simulink model "LowPassRC_Filter"  (R2021a)
settings: Solver=FixedStepAuto  StartTime=0.0  StopTime=10.0  FixedStep=0.0001  RelTol=1e-3
libraries: simulink x1
settings Model: Creator=F Octopus The Grey  LastModifiedBy=F Octopus The Grey

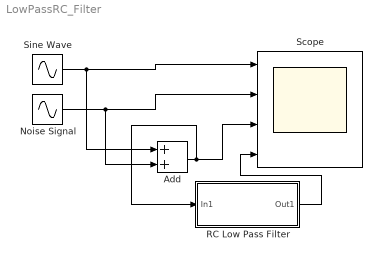
== system LowPassRC_Filter ==
  Add : Sum
  Noise Signal : Sin  Amplitude=5  Frequency=10  SampleTime=0
  RC Low Pass Filter : Subsystem
  Scope : Scope  NumInputPorts=4
  Sine Wave : Sin  Amplitude=50  SampleTime=0
  wires:
  Sine Wave/1 -> Add/1, Scope/1
  Noise Signal/1 -> Add/2, Scope/2
  Add/1 -> RC Low Pass Filter/1(In1), Scope/3
  RC Low Pass Filter/1(Out1) -> Scope/4

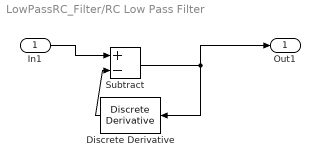
== system LowPassRC_Filter/RC Low Pass Filter ==
  In1 : Inport
  Discrete Derivative : simulink/Discrete/Discrete Derivative  gainval=1.0  ICPrevScaledInput=0.0  OutMin=[]  OutMax=[]  OutDataType=fixdt(1, 16)  OutScaling=2^-10  DoSatur=off
  Subtract : Sum  Inputs=+-
  Out1 : Outport
  wires:
  In1/1 -> Subtract/1
  Subtract/1 -> Discrete Derivative/1, Out1/1
  Discrete Derivative/1 -> Subtract/2
